simulink model "Model"  (R2015a)
settings: Solver=ode45  StartTime=0.0  StopTime=10.0  RelTol=1e-3
settings Model: Creator=laragoxhaj  LastModifiedBy=solvie

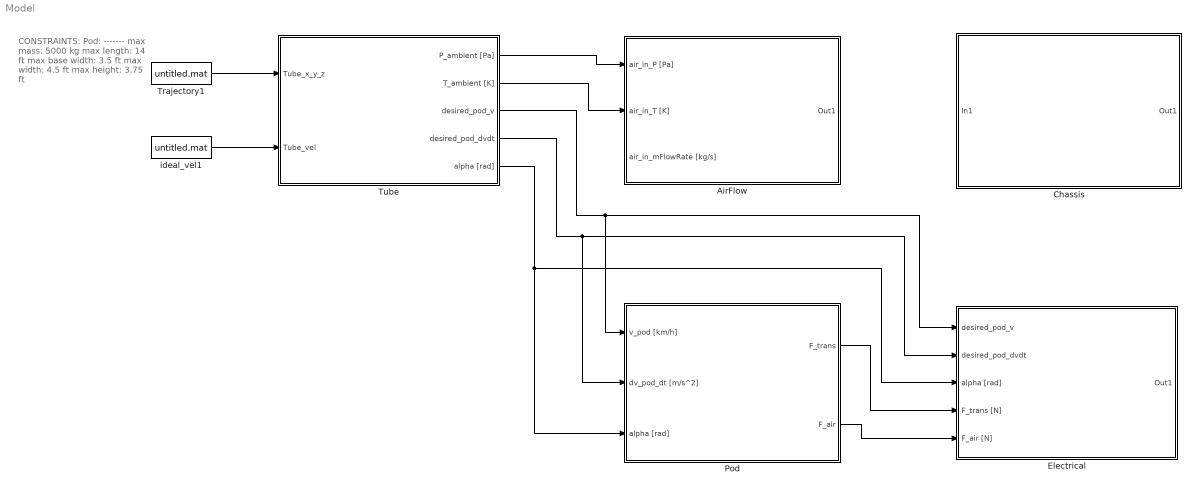
== system Model ==
  note: CONSTRAINTS:
      |
      | Pod:
      | -------
      | max mass:		5000 kg
      | max length:		14 ft
      | max base width:	3.5 ft
      | max width:		4.5 ft
      | max height:		3.75 ft
  AirFlow : Subsystem
  Chassis : Subsystem
  Electrical : Subsystem
  Pod : Subsystem
  Trajectory1 : FromFile  SampleTime=0
  Tube : Subsystem
  ideal_vel1 : FromFile  SampleTime=0
  wires:
  Tube/1(P_ambient [Pa]) -> AirFlow/1(air_in_P [Pa])
  Tube/2(T_ambient [K]) -> AirFlow/2(air_in_T [K])
  Pod/2(F_air) -> Electrical/5(F_air [N])
  Pod/1(F_trans) -> Electrical/4(F_trans [N])
  Tube/3(desired_pod_v) -> Pod/1(v_pod [km/h]), Electrical/1(desired_pod_v)
  Tube/4(desired_pod_dvdt) -> Pod/2(dv_pod_dt [m/s^2]), Electrical/2(desired_pod_dvdt)
  Tube/5(alpha [rad]) -> Electrical/3(alpha [rad]), Pod/3(alpha [rad])
  Trajectory1/1 -> Tube/1(Tube_x_y_z)
  ideal_vel1/1 -> Tube/2(Tube_vel)

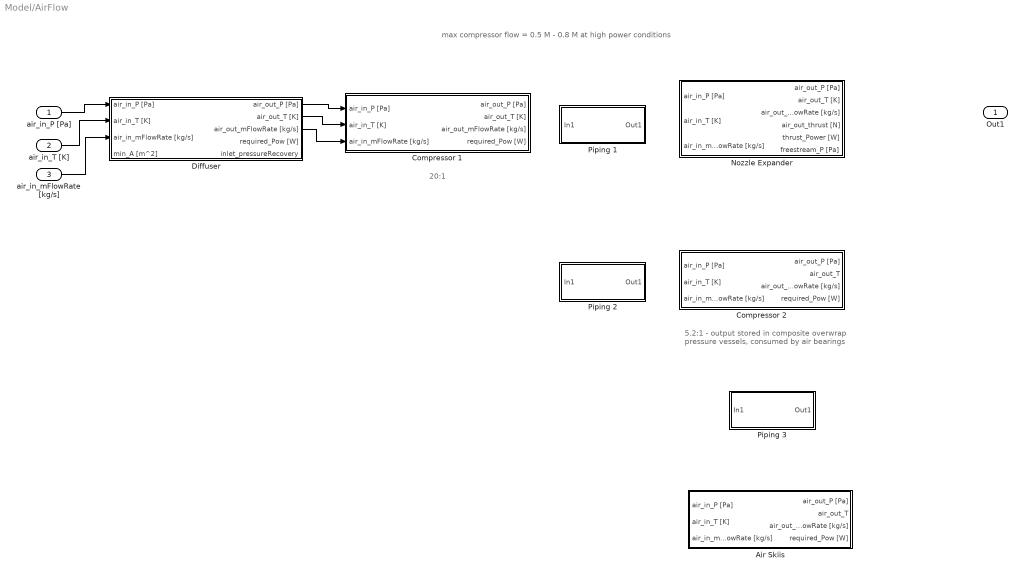
== system Model/AirFlow ==
  note: 20:1
  note: max compressor flow = 0.5 M - 0.8 M at high power conditions
  note: 5.2:1 - output stored in composite overwrap
      | pressure vessels, consumed by air bearings
  air_in_P [Pa] : Inport
  air_in_T [K] : Inport  Port=2
  air_in_mFlowRate [kg/s] : Inport  Port=3
  Air Skiis : Subsystem
  Compressor 1 : Subsystem
  Compressor 2 : Subsystem
  Diffuser : Subsystem
  Nozzle Expander : Subsystem
  Piping 1 : Subsystem
  Piping 2 : Subsystem
  Piping 3 : Subsystem
  Out1 : Outport
  wires:
  Diffuser/1(air_out_P [Pa]) -> Compressor 1/1(air_in_P [Pa])
  Diffuser/2(air_out_T [K]) -> Compressor 1/2(air_in_T [K])
  Diffuser/3(air_out_mFlowRate [kg/s]) -> Compressor 1/3(air_in_mFlowRate [kg/s])
  air_in_P [Pa]/1 -> Diffuser/1(air_in_P [Pa])
  air_in_T [K]/1 -> Diffuser/2(air_in_T [K])
  air_in_mFlowRate [kg/s]/1 -> Diffuser/3(air_in_mFlowRate [kg/s])

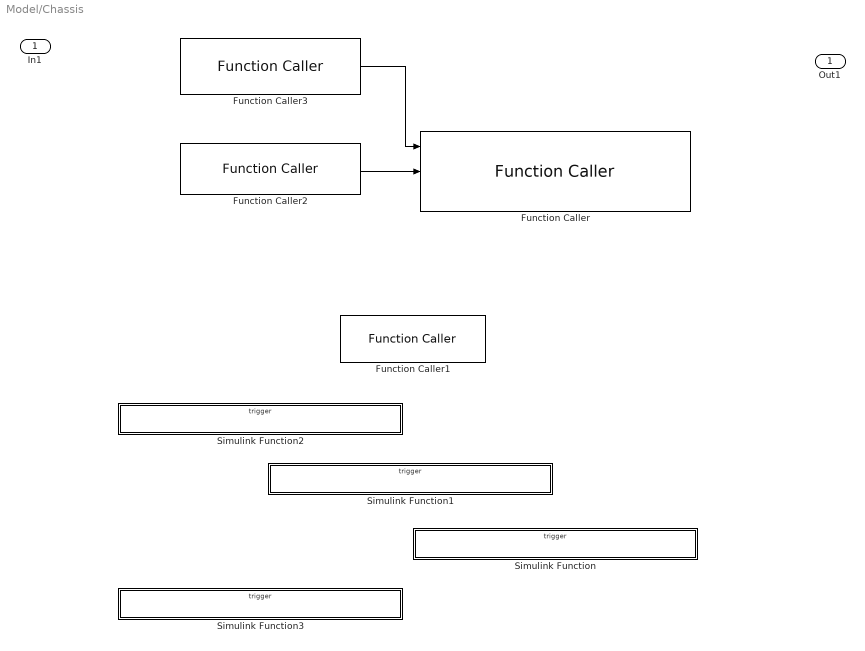
== system Model/Chassis ==
  In1 : Inport
  Function Caller : FunctionCaller  FunctionPrototype=bypass_air_mFlowRate = f(air_density,bypass_A,pod_v)
  Function Caller1 : FunctionCaller  FunctionPrototype=released_Q = f(max_Q,effectiveness)
  Function Caller2 : FunctionCaller  FunctionPrototype=bypass_A = f(tube_r,pod_r)
  Function Caller3 : FunctionCaller  FunctionPrototype=air_density = f(ambient_P,R_air,ambient_T)
  Simulink Function : Subsystem  TreatAsAtomicUnit=on
  Simulink Function1 : Subsystem  TreatAsAtomicUnit=on
  Simulink Function2 : Subsystem  TreatAsAtomicUnit=on
  Simulink Function3 : Subsystem  TreatAsAtomicUnit=on
  Out1 : Outport
  wires:
  Function Caller2/1 -> Function Caller/2
  Function Caller3/1 -> Function Caller/1

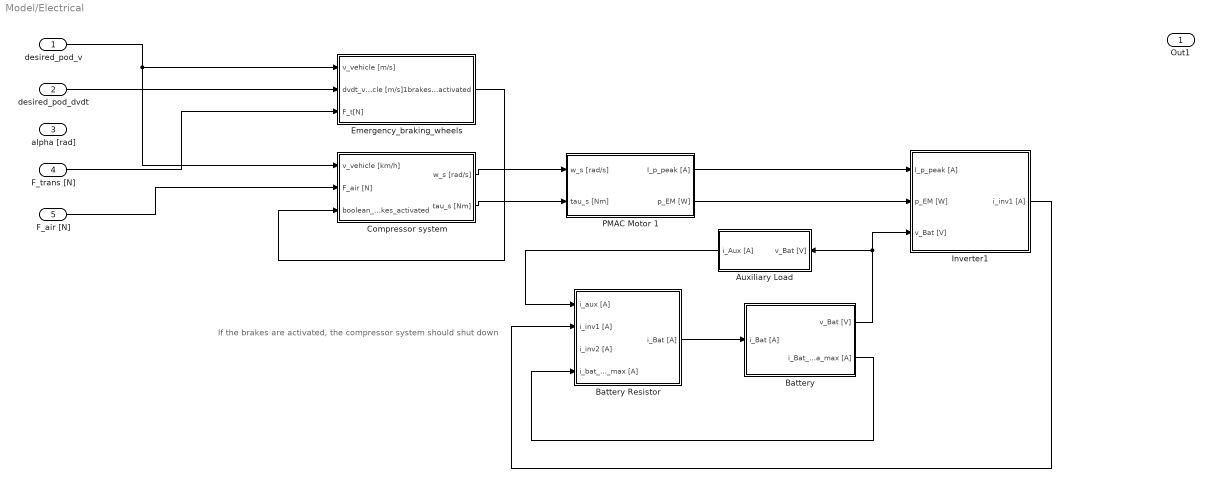
== system Model/Electrical ==
  note: If the brakes are activated, the compressor system should shut down
  desired_pod_v : Inport
  desired_pod_dvdt : Inport  Port=2
  alpha [rad] : Inport  Port=3
  F_trans [N] : Inport  Port=4
  F_air [N] : Inport  Port=5
  Auxiliary Load : Subsystem
  Battery : Subsystem
  Battery Resistor : Subsystem
  Compressor system : Subsystem
  Emergency_braking_wheels : Subsystem
  Inverter1 : Subsystem
  PMAC Motor 1 : Subsystem
  Out1 : Outport
  wires:
  Compressor system/1(w_s [rad/s]) -> PMAC Motor 1/1(w_s [rad/s])
  Compressor system/2(tau_s [Nm]) -> PMAC Motor 1/2(tau_s [Nm])
  PMAC Motor 1/1(I_p_peak [A]) -> Inverter1/1(I_p_peak [A])
  PMAC Motor 1/2(p_EM [W]) -> Inverter1/2(p_EM [W])
  Auxiliary Load/1(i_Aux [A]) -> Battery Resistor/1(i_aux [A])
  Battery Resistor/1(i_Bat [A]) -> Battery/1(i_Bat [A])
  Battery/1(v_Bat [V]) -> Inverter1/3(v_Bat [V]), Auxiliary Load/1(v_Bat [V])
  Battery/2(i_Bat_cha_max [A]) -> Battery Resistor/4(i_bat_cha_max [A])
  Inverter1/1(i_inv1 [A]) -> Battery Resistor/2(i_inv1 [A])
  desired_pod_v/1 -> Compressor system/1(v_vehicle [km/h]), Emergency_braking_wheels/1(v_vehicle [m/s])
  F_trans [N]/1 -> Emergency_braking_wheels/3(F_t[N])
  F_air [N]/1 -> Compressor system/2(F_air [N])
  desired_pod_dvdt/1 -> Emergency_braking_wheels/2(dvdt_vehicle [m/s]1)
  Emergency_braking_wheels/1(brakes_activated) -> Compressor system/3(boolean_brakes_activated)

== system Model/Pod ==
  v_pod [km/h] : Inport
  dv_pod_dt [m/s^2] : Inport  Port=2
  alpha [rad] : Inport  Port=3
  F_trans : Outport
  F_air : Outport  Port=2

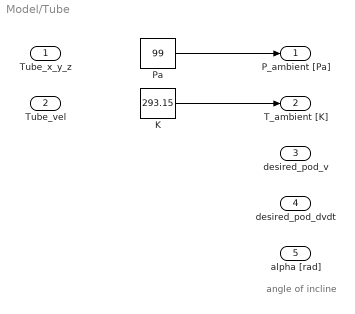
== system Model/Tube ==
  note: angle of incline
  Tube_x_y_z : Inport
  Tube_vel : Inport  Port=2
  K : Constant  Value=293.15
  Pa : Constant  Value=99
  P_ambient [Pa] : Outport
  T_ambient [K] : Outport  Port=2
  desired_pod_v : Outport  Port=3
  desired_pod_dvdt : Outport  Port=4
  alpha [rad] : Outport  Port=5
  wires:
  Pa/1 -> P_ambient [Pa]/1
  K/1 -> T_ambient [K]/1

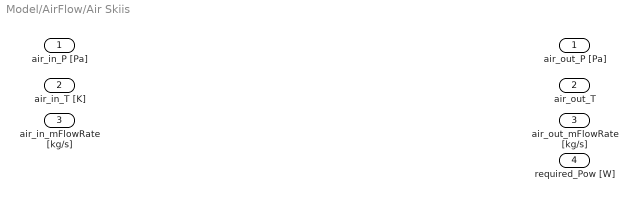
== system Model/AirFlow/Air Skiis ==
  air_in_P [Pa] : Inport
  air_in_T [K] : Inport  Port=2
  air_in_mFlowRate [kg/s] : Inport  Port=3
  air_out_P [Pa] : Outport
  air_out_T : Outport  Port=2
  air_out_mFlowRate [kg/s] : Outport  Port=3
  required_Pow [W] : Outport  Port=4

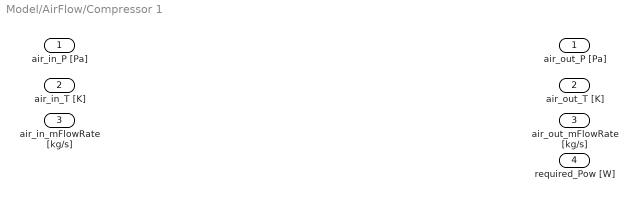
== system Model/AirFlow/Compressor 1 ==
  air_in_P [Pa] : Inport
  air_in_T [K] : Inport  Port=2
  air_in_mFlowRate [kg/s] : Inport  Port=3
  air_out_P [Pa] : Outport
  air_out_T [K] : Outport  Port=2
  air_out_mFlowRate [kg/s] : Outport  Port=3
  required_Pow [W] : Outport  Port=4

== system Model/AirFlow/Compressor 2 ==
  air_in_P [Pa] : Inport
  air_in_T [K] : Inport  Port=2
  air_in_mFlowRate [kg/s] : Inport  Port=3
  air_out_P [Pa] : Outport
  air_out_T : Outport  Port=2
  air_out_mFlowRate [kg/s] : Outport  Port=3
  required_Pow [W] : Outport  Port=4

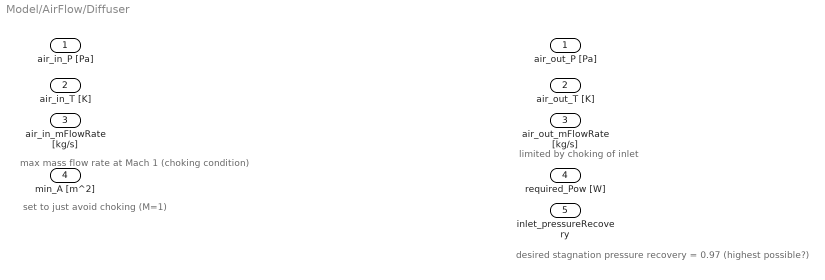
== system Model/AirFlow/Diffuser ==
  note: set to just avoid choking (M=1)
  note: desired stagnation pressure recovery = 0.97 (highest possible?)
  note: limited by choking of inlet
  note: max mass flow rate at Mach 1 (choking condition)
  air_in_P [Pa] : Inport
  air_in_T [K] : Inport  Port=2
  air_in_mFlowRate [kg/s] : Inport  Port=3
  min_A [m^2] : Inport  Port=4
  air_out_P [Pa] : Outport
  air_out_T [K] : Outport  Port=2
  air_out_mFlowRate [kg/s] : Outport  Port=3
  required_Pow [W] : Outport  Port=4
  inlet_pressureRecovery : Outport  Port=5

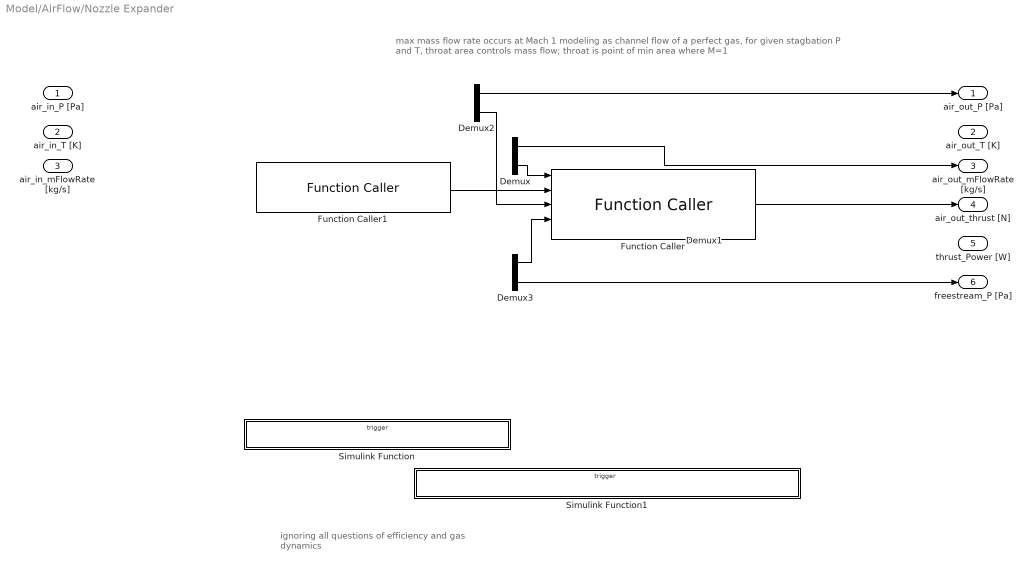
== system Model/AirFlow/Nozzle Expander ==
  note: ignoring all questions of efficiency and gas
      | dynamics
  note: max mass flow rate occurs at Mach 1
      | modeling as channel flow of a perfect gas, for given stagbation P and T, throat area controls mass flow; throat is point of min area where M=1
  air_in_P [Pa] : Inport
  air_in_T [K] : Inport  Port=2
  air_in_mFlowRate [kg/s] : Inport  Port=3
  Demux{,1..3} (4 alike) : Demux  Outputs=2
  Function Caller : FunctionCaller  FunctionPrototype=thrust = rocketEq(expulsion_mFlowRate,relative_v,exit_P,freestream_P,exit_A)
  Function Caller1 : FunctionCaller  FunctionPrototype=exhaust_v = velocity_exhaust(stagnation_T,gamma)
  Simulink Function : Subsystem  TreatAsAtomicUnit=on
  Simulink Function1 : Subsystem  TreatAsAtomicUnit=on
  air_out_P [Pa] : Outport
  air_out_T [K] : Outport  Port=2
  air_out_mFlowRate [kg/s] : Outport  Port=3
  air_out_thrust [N] : Outport  Port=4
  thrust_Power [W] : Outport  Port=5
  freestream_P [Pa] : Outport  Port=6
  wires:
  Function Caller1/1 -> Function Caller/2
  Demux/1 -> air_out_mFlowRate [kg/s]/1
  Demux/2 -> Function Caller/1
  Demux2/2 -> Function Caller/3
  Demux2/1 -> air_out_P [Pa]/1
  Demux3/1 -> Function Caller/4
  Demux3/2 -> freestream_P [Pa]/1
  Function Caller/1 -> air_out_thrust [N]/1

== system Model/AirFlow/Piping 1 ==
  In1 : Inport
  Out1 : Outport
  wires:
  In1/1 -> Out1/1

== system Model/AirFlow/Piping 2 ==
  In1 : Inport
  Out1 : Outport
  wires:
  In1/1 -> Out1/1

== system Model/AirFlow/Piping 3 ==
  In1 : Inport
  Out1 : Outport
  wires:
  In1/1 -> Out1/1

== system Model/Chassis/Simulink Function ==
  f : TriggerPort  TriggerType=function-call  IsSimulinkFunction=on  FunctionName=f
  Product : Product  Inputs=3
  air_density : ArgIn  DisableCoverage=on  ArgumentName=air_density
  bypass_A : ArgIn  DisableCoverage=on  Port=2  ArgumentName=bypass_A
  pod_v : ArgIn  DisableCoverage=on  Port=3  ArgumentName=pod_v
  bypass_air_mFlowRate : ArgOut  DisableCoverage=on  ArgumentName=bypass_air_mFlowRate
  wires:
  air_density/1 -> Product/1
  bypass_A/1 -> Product/2
  pod_v/1 -> Product/3
  Product/1 -> bypass_air_mFlowRate/1

== system Model/Chassis/Simulink Function1 ==
  heat : TriggerPort  TriggerType=function-call  IsSimulinkFunction=on  FunctionName=f
  Product : Product
  air_density : ArgIn  DisableCoverage=on  ArgumentName=max_Q
  bypass_A : ArgIn  DisableCoverage=on  Port=2  ArgumentName=effectiveness
  bypass_air_mFlowRate : ArgOut  DisableCoverage=on  ArgumentName=released_Q
  wires:
  air_density/1 -> Product/1
  bypass_A/1 -> Product/2
  Product/1 -> bypass_air_mFlowRate/1

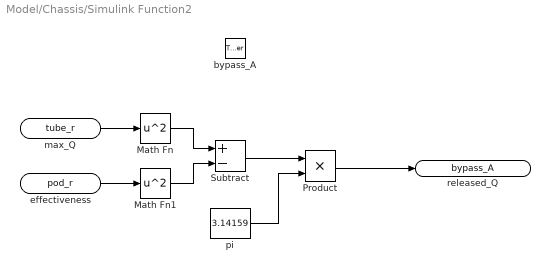
== system Model/Chassis/Simulink Function2 ==
  bypass_A : TriggerPort  TriggerType=function-call  IsSimulinkFunction=on  FunctionName=f
  Math Fn : Math  Operator=square  SaturateOnIntegerOverflow=on
  Math Fn1 : Math  Operator=square  SaturateOnIntegerOverflow=on
  Product : Product
  Subtract : Sum  Inputs=+-
  pi : Constant  Value=3.14159
  max_Q : ArgIn  DisableCoverage=on  ArgumentName=tube_r
  effectiveness : ArgIn  DisableCoverage=on  Port=2  ArgumentName=pod_r
  released_Q : ArgOut  DisableCoverage=on  ArgumentName=bypass_A
  wires:
  max_Q/1 -> Math Fn/1
  effectiveness/1 -> Math Fn1/1
  Math Fn/1 -> Subtract/1
  Math Fn1/1 -> Subtract/2
  Subtract/1 -> Product/1
  pi/1 -> Product/2
  Product/1 -> released_Q/1

== system Model/Chassis/Simulink Function3 ==
  f : TriggerPort  TriggerType=function-call  IsSimulinkFunction=on  FunctionName=f
  Divide : Product  Inputs=*/
  Product : Product
  ambient_P : ArgIn  DisableCoverage=on  ArgumentName=ambient_P
  R_air : ArgIn  DisableCoverage=on  Port=2  ArgumentName=R_air
  ambient_T : ArgIn  DisableCoverage=on  Port=3  ArgumentName=ambient_T
  air_density : ArgOut  DisableCoverage=on  ArgumentName=air_density
  wires:
  R_air/1 -> Product/1
  ambient_T/1 -> Product/2
  ambient_P/1 -> Divide/1
  Divide/1 -> air_density/1
  Product/1 -> Divide/2

== system Model/Electrical/Auxiliary Load ==
  v_Bat [V] : Inport
  i_Aux [A] : Outport
  wires:
  v_Bat [V]/1 -> i_Aux [A]/1

== system Model/Electrical/Battery ==
  i_Bat [A] : Inport
  v_Bat [V] : Outport
  i_Bat_cha_max [A] : Outport  Port=2

== system Model/Electrical/Battery Resistor ==
  i_aux [A] : Inport
  i_inv1 [A] : Inport  Port=2
  i_inv2 [A] : Inport  Port=3
  i_bat_cha_max [A] : Inport  Port=4
  i_Bat [A] : Outport

== system Model/Electrical/Compressor system ==
  v_vehicle [km/h] : Inport
  F_air [N] : Inport  Port=2
  boolean_brakes_activated : Inport  Port=3
  w_s [rad/s] : Outport
  tau_s [Nm] : Outport  Port=2

== system Model/Electrical/Emergency_braking_wheels ==
  v_vehicle [m/s] : Inport
  dvdt_vehicle [m/s]1 : Inport  Port=2
  F_t[N] : Inport  Port=3
  brakes_activated : Outport

== system Model/Electrical/Inverter1 ==
  I_p_peak [A] : Inport
  p_EM [W] : Inport  Port=2
  v_Bat [V] : Inport  Port=3
  i_inv1 [A] : Outport

== system Model/Electrical/PMAC Motor 1 ==
  w_s [rad/s] : Inport
  tau_s [Nm] : Inport  Port=2
  I_p_peak [A] : Outport
  p_EM [W] : Outport  Port=2

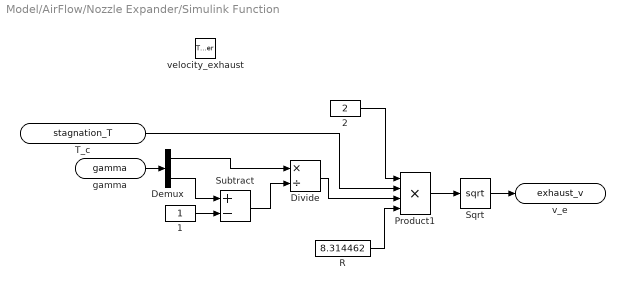
== system Model/AirFlow/Nozzle Expander/Simulink Function ==
  velocity_exhaust : TriggerPort  TriggerType=function-call  IsSimulinkFunction=on  FunctionName=velocity_exhaust
  1 : Constant
  2 : Constant  Value=2
  Demux : Demux  Outputs=2
  Divide : Product  Inputs=*/
  Product1 : Product  Inputs=4
  R : Constant  Value=8.314462
  Sqrt : Sqrt  SaturateOnIntegerOverflow=on
  Subtract : Sum  Inputs=+-
  T_c : ArgIn  DisableCoverage=on  ArgumentName=stagnation_T
  gamma : ArgIn  DisableCoverage=on  Port=2  ArgumentName=gamma
  v_e : ArgOut  DisableCoverage=on  ArgumentName=exhaust_v
  wires:
  T_c/1 -> Product1/2
  Product1/1 -> Sqrt/1
  Sqrt/1 -> v_e/1
  2/1 -> Product1/1
  R/1 -> Product1/4
  Divide/1 -> Product1/3
  1/1 -> Subtract/2
  Demux/1 -> Divide/1
  gamma/1 -> Demux/1
  Demux/2 -> Subtract/1
  Subtract/1 -> Divide/2

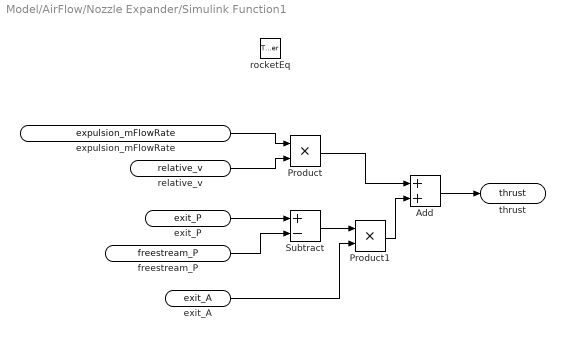
== system Model/AirFlow/Nozzle Expander/Simulink Function1 ==
  rocketEq : TriggerPort  TriggerType=function-call  IsSimulinkFunction=on  FunctionName=rocketEq
  Add : Sum
  Product : Product
  Product1 : Product
  Subtract : Sum  Inputs=+-
  expulsion_mFlowRate : ArgIn  DisableCoverage=on  ArgumentName=expulsion_mFlowRate
  relative_v : ArgIn  DisableCoverage=on  Port=2  ArgumentName=relative_v
  exit_P : ArgIn  DisableCoverage=on  Port=3  ArgumentName=exit_P
  freestream_P : ArgIn  DisableCoverage=on  Port=4  ArgumentName=freestream_P
  exit_A : ArgIn  DisableCoverage=on  Port=5  ArgumentName=exit_A
  thrust : ArgOut  DisableCoverage=on  ArgumentName=thrust
  wires:
  relative_v/1 -> Product/2
  expulsion_mFlowRate/1 -> Product/1
  Product/1 -> Add/1
  Product1/1 -> Add/2
  Add/1 -> thrust/1
  exit_A/1 -> Product1/2
  exit_P/1 -> Subtract/1
  freestream_P/1 -> Subtract/2
  Subtract/1 -> Product1/1
